simulink model "Noise"  (Simulink 10.3)
settings: Solver=FixedStepDiscrete  StartTime=0.0  StopTime=2000.0  RelTol=1e-3
libraries: dsp_blocks x10, simulink x1
settings Model: Creator=nathanalemayehu  LastModifiedBy=nathanalemayehu
settings SolverCC: AlgebraicLoopSolver=Auto
settings DataIOCC: SaveFormat=Dataset  SignalLoggingSaveFormat=Dataset  ReturnWorkspaceOutputs=on
settings OptimizationCC: ExpressionDepthLimit=128  LifeSpan=auto
settings DebuggingCC: UnderspecifiedInitializationDetection=Simplified  MergeDetectMultiDrivingBlocksExec=error  FcnCallInpInsideContextMsg=error  StateNameClashWarn=none  SFUnexpectedBacktrackingDiag=error  SFNoUnconditionalDefaultTransitionDiag=error  SFExecutionAtInitializationDiag=warning  SFMachineParentedDataDiag=error  ArithmeticOperatorsInVariantConditions=error
settings HardwareCC: ProdBitPerPointer=64  ProdBitPerSizeT=64  ProdBitPerPtrDiffT=64  ProdLargestAtomicFloat=Float  ProdIntDivRoundTo=Zero  ProdEndianess=LittleEndian  ProdWordSize=64  ProdHWDeviceType=Intel->x86-64 (Windows64)
settings ModelReferenceCC: PropagateSignalLabelsOutOfModel=on
settings SFSimCC: SimUseLocalCustomCode=on  CustomCodeUndefinedFunction=FilterOut
settings RTWCC: RTWUseLocalCustomCode=on
settings CodeAppCC: StateflowObjectComments=off
settings GRTTargetCC: TargetLangStandard=C99 (ISO)  CombineOutputUpdateFcns=on  GRTInterface=off
settings ConfigComp: CovMetricSettings=dwe  CovSaveCumulativeToWorkspaceVar=off  CovSaveSingleToWorkspaceVar=off  CovExternalEMLEnable=on

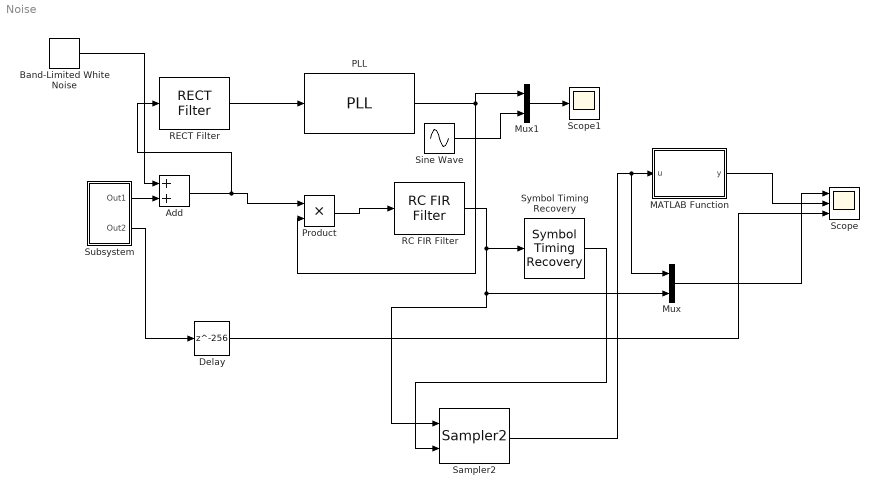
== system Noise ==
  Add : Sum
  Band-Limited White Noise : simulink/Sources/Band-Limited White Noise  Cov=[0.01]  Ts=1  seed=[23341]
  Delay : Delay  DelayLength=256
  MATLAB Function : MATLAB Function  TreatAsAtomicUnit=on
  Mux : Mux  Inputs=2
  Mux1 : Mux  Inputs=2
  PLL : dsp_blocks/Timing /PLL  freq=0.05  freq_out=0.1  phi=0  amp=2  xi=1  K=2  T=200
  Product : Product
  RC FIR Filter : dsp_blocks/Filters/RC FIR Filter  period=50  beta=0.5  root=on  filt_len=512  win_type=on
  RECT Filter : dsp_blocks/Filters/RECT Filter  f0=0.03  f1=0.07  filt_len=80
  Sampler2 : dsp_blocks/Conversions/Sampler2
  Scope : Scope  NumInputPorts=3
  Scope1 : Scope
  Sine Wave : Sin  Frequency=2*pi*0.05  SampleTime=0
  Subsystem : Subsystem
  Symbol Timing Recovery : dsp_blocks/Timing /Symbol Timing Recovery  T=50  Tl=1000  tadj=-1
  wires:
  PLL/1 -> Product/2, Mux1/1
  Sampler2/1 -> Mux/1, MATLAB Function/1(u)
  RECT Filter/1 -> PLL/1
  Mux1/1 -> Scope1/1
  Sine Wave/1 -> Mux1/2
  Product/1 -> RC FIR Filter/1
  Symbol Timing Recovery/1 -> Sampler2/2
  Delay/1 -> Scope/3
  RC FIR Filter/1 -> Sampler2/1, Mux/2, Symbol Timing Recovery/1
  MATLAB Function/1(y) -> Scope/2
  Subsystem/2(Out2) -> Delay/1
  Mux/1 -> Scope/1
  Subsystem/1(Out1) -> Add/2
  Add/1 -> RECT Filter/1, Product/1
  Band-Limited White Noise/1 -> Add/1

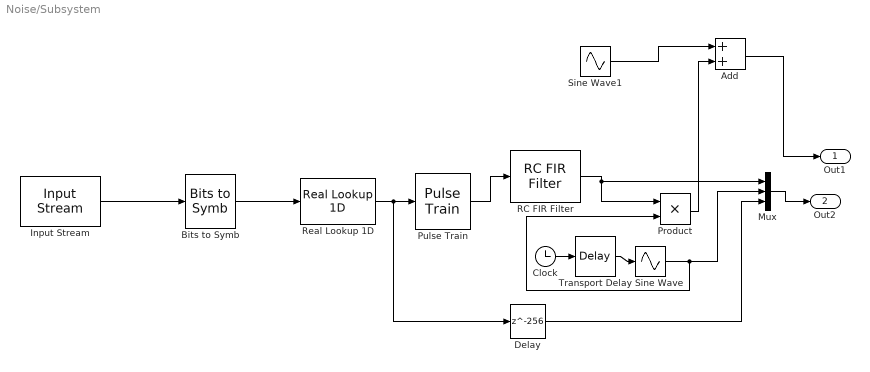
== system Noise/Subsystem ==
  Add : Sum
  Bits to Symb : dsp_blocks/Conversions/Bits to Symb
  Clock : Clock
  Delay : Delay  DelayLength=256
  Input Stream : dsp_blocks/Sources//Sinks/Input Stream  period=50  width=1  fname=rand.mat
  Mux : Mux  Inputs=3
  Product : Product
  Pulse Train : dsp_blocks/Conversions/Pulse Train  period=50
  RC FIR Filter : dsp_blocks/Filters/RC FIR Filter  period=50  beta=0.5  root=on  filt_len=512  win_type=on
  Real Lookup 1D : dsp_blocks/Conversions/Real Lookup 1D  table=[-1 1]
  Sine Wave : Sin  TimeSource=Use external signal  Frequency=2*pi*0.1  SampleTime=0
  Sine Wave1 : Sin  Amplitude=0.05  Frequency=2*pi*0.05  SampleTime=0
  Transport Delay : TransportDelay
  Out1 : Outport
  Out2 : Outport  Port=2
  wires:
  Input Stream/1 -> Bits to Symb/1
  Bits to Symb/1 -> Real Lookup 1D/1
  Product/1 -> Add/2
  Sine Wave/1 -> Mux/2, Product/2
  Pulse Train/1 -> RC FIR Filter/1
  Mux/1 -> Out2/1
  Real Lookup 1D/1 -> Delay/1, Pulse Train/1
  Delay/1 -> Mux/3
  RC FIR Filter/1 -> Product/1, Mux/1
  Clock/1 -> Transport Delay/1
  Transport Delay/1 -> Sine Wave/1
  Sine Wave1/1 -> Add/1
  Add/1 -> Out1/1

== matlab function MATLAB Function ==
  data: u input double; y output double
function y = fcn(u)
if(u > 0),
    y = 1;
else 
    y = 0;
end
